simulink model "lab3simulink"  (R2019b)
settings: Solver=ode45  StartTime=0.0  StopTime=0.2  RelTol=1e-3
settings Model: Creator=wesle  LastModifiedBy=wesle
settings OptimizationCC: BooleanDataType=off

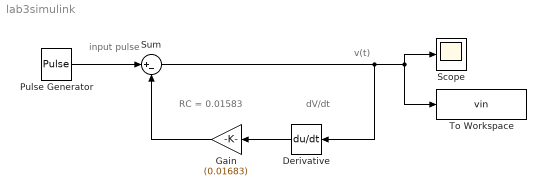
== system lab3simulink ==
  note: v(t)
  note: dV/dt
  note: RC = 0.01583
  note: input pulse
  Derivative : Derivative
  Gain : Gain  Gain=(0.01683)
  Pulse Generator : DiscretePulseGenerator  PulseType=Time based  Amplitude=60  Period=1000  PulseWidth=0.00016
  Scope : Scope
  Sum : Sum  Inputs=|+-
  To Workspace : ToWorkspace  VariableName=vin  SampleTime=-1
  wires:
  Sum/1 -> Derivative/1, To Workspace/1, Scope/1
  Pulse Generator/1 -> Sum/1
  Derivative/1 -> Gain/1
  Gain/1 -> Sum/2
